simulink model "Fig5_Control_RLcurrent_OhmsLaw"  (R2022a)
settings: Solver=FixedStepAuto  StartTime=0.0  StopTime=0.4  FixedStep=1e-4  RelTol=1e-3
InitFcn:
  | RLCurcuitParam
StartFcn:
  | RLCurcuitParam
values from neighbouring files (symbols this model uses):
  L = 4e-3    (= 0.004)    [Fig17_drawBodeCPminusP.m]    (also in KpKiDesign.m; RLCurcuitParam.m)
  R = 0.1    [Fig17_drawBodeCPminusP.m]    (also in KpKiDesign.m; RLCurcuitParam.m)
settings Model: Creator=r720r  LastModifiedBy=r720r

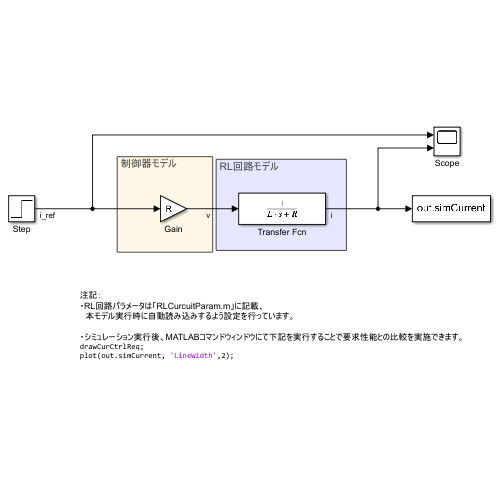
[thumbnail: Simulink's stored preview of the top-level diagram]
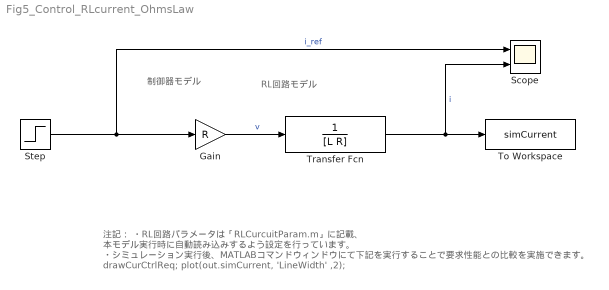
== system Fig5_Control_RLcurrent_OhmsLaw ==
  note: 注記：
      | ・RL回路パラメータは「RLCurcuitParam.m」に記載、
      | 本モデル実行時に自動読み込みするよう設定を行っています。
      |
      | ・シミュレーション実行後、MATLABコマンドウィンドウにて下記を実行することで要求性能との比較を実施できます。
      | drawCurCtrlReq;
      | plot(out.simCurrent, 'LineWidth' ,2);
  note: RL回路モデル
  note: 制御器モデル
  Gain : Gain  Gain=R
  Scope : Scope  NumInputPorts=2
  Step : Step  Time=0  SampleTime=0
  To Workspace : ToWorkspace  VariableName=simCurrent  SaveFormat=Timeseries  SampleTime=-1
  Transfer Fcn : TransferFcn  Denominator=[L R]
  wires:
  Step/1 -> Scope/1, Gain/1  "i_ref"
  Transfer Fcn/1 -> To Workspace/1, Scope/2  "i"
  Gain/1 -> Transfer Fcn/1  "v"
